simulink model "Motor_Servo_Final"  (R2026a)
settings: Solver=VariableStepAuto  StopTime=10
values from neighbouring files (symbols this model uses):
  b = 0.1    [parameters.m]
  J = 0.01    [parameters.m]
  K = Ka(1:2)    [observer_design.m]    (also in servo_controller.m; state_feedback.m = place(A,B,desired_poles))
  Ke = 0.01    [parameters.m]
  Ki = -Ka(3)    [observer_design.m]    (also in servo_controller.m = Ka(3))
  Kt = 0.01    [parameters.m]
  L = 0.5    [observer_design.m]    (also in parameters.m)
  R = 1    [parameters.m]
settings Model: Creator=DELL  LastModifiedBy=DELL

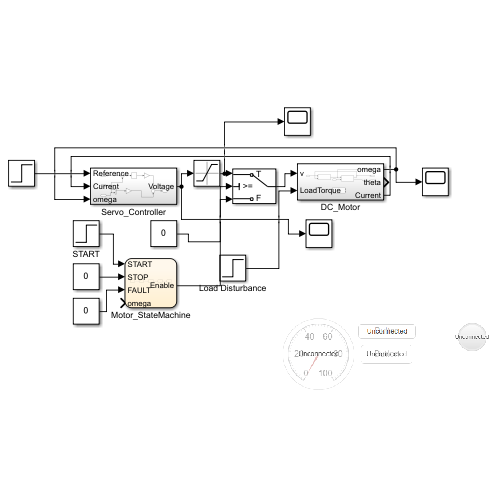
[thumbnail: Simulink's stored preview of the top-level diagram]
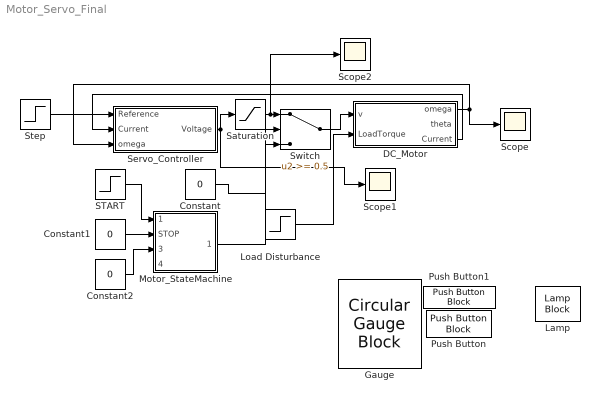
== system Motor_Servo_Final ==
  Constant : Constant  Value=0
  Constant1 : Constant  Value=0
  Constant2 : Constant  Value=0
  DC_Motor : Subsystem
  Gauge : CircularGaugeBlock  FontColor=[0.0, 0.0, 0.0]
  Lamp : LampBlock  LabelPosition=Hide  DefaultColor=[192.0, 192.0, 192.0]
  Load Disturbance : Step  Time=2  FinalValue=0.02  SampleTime=0
  Motor_StateMachine : Stateflow chart  TreatAsAtomicUnit=on
  Push Button : PushButtonBlock  IconOnColor=[0.0, 0.39215686274509803, 0.0]  IconOffColor=[0.0, 1.0, 0.0]
  Push Button1 : PushButtonBlock  IconOnColor=[0.0, 0.39215686274509803, 0.0]  IconOffColor=[0.0, 1.0, 0.0]
  START : Step  Time=0  SampleTime=0
  Saturation : Saturate  UpperLimit=220  LowerLimit=-220
  Scope : Scope
      settings: ActiveDisplayYMinimum=-0.091246608325466383  ActiveDisplayYMaximum=1.905925597827455
  Scope1 : Scope
      settings: ActiveDisplayYMinimum=-1002.8339969118642  ActiveDisplayYMaximum=2013.0889387942134
  Scope2 : Scope
      settings: ActiveDisplayYMinimum=-27.499999999999993  ActiveDisplayYMaximum=247.5  DataLoggingVariableName=ScopeData2
  Servo_Controller : Subsystem
  Step : Step  Time=0  FinalValue=10  SampleTime=0
  Switch : Switch  Threshold=0.5  SaturateOnIntegerOverflow=off  InputSameDT=off
  wires:
  DC_Motor/1(omega) -> Scope/1, Servo_Controller/3(omega)
  Load Disturbance/1 -> DC_Motor/2(LoadTorque)
  DC_Motor/3(Current) -> Servo_Controller/2(Current)
  Constant/1 -> Switch/3
  START/1 -> Motor_StateMachine/1(START)
  Constant1/1 -> Motor_StateMachine/2(STOP)
  Constant2/1 -> Motor_StateMachine/3(FAULT)
  Step/1 -> Servo_Controller/1(Reference)
  Motor_StateMachine/1(Enable) -> Switch/2
  Switch/1 -> DC_Motor/1(v)
  Servo_Controller/1(Voltage) -> Saturation/1, Scope1/1
  Saturation/1 -> Scope2/1, Switch/1

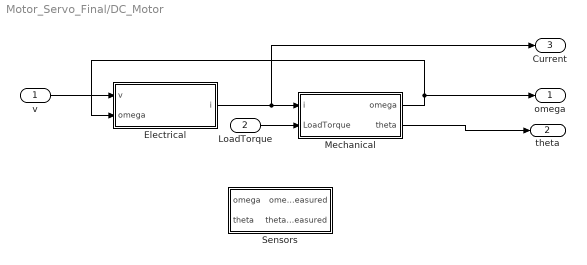
== system Motor_Servo_Final/DC_Motor ==
  v : Inport
  LoadTorque : Inport  Port=2
  Electrical : Subsystem
  Mechanical : Subsystem
  Sensors : Subsystem
  omega : Outport
  theta : Outport  Port=2
  Current : Outport  Port=3
  wires:
  v/1 -> Electrical/1(v)
  Mechanical/1(omega) -> Electrical/2(omega), omega/1
  Mechanical/2(theta) -> theta/1
  LoadTorque/1 -> Mechanical/2(LoadTorque)
  Electrical/1(i) -> Current/1, Mechanical/1(i)

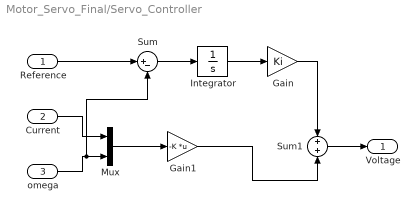
== system Motor_Servo_Final/Servo_Controller ==
  Reference : Inport
  Current : Inport  Port=2
  omega : Inport  Port=3
  Gain : Gain  Gain=Ki
  Gain1 : Gain  Gain=-K  Multiplication=Matrix(K*u)
  Integrator : Integrator
  Mux : Mux  Inputs=2
  Sum : Sum  Inputs=|+-
  Sum1 : Sum
  Voltage : Outport
  wires:
  omega/1 -> Sum/2, Mux/2
  Current/1 -> Mux/1
  Reference/1 -> Sum/1
  Sum/1 -> Integrator/1
  Integrator/1 -> Gain/1
  Mux/1 -> Gain1/1
  Gain/1 -> Sum1/1
  Gain1/1 -> Sum1/2
  Sum1/1 -> Voltage/1

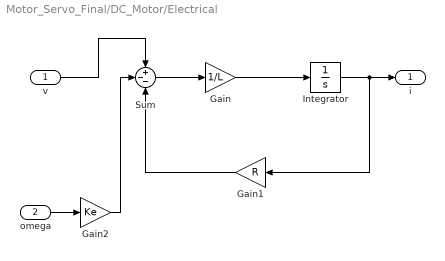
== system Motor_Servo_Final/DC_Motor/Electrical ==
  v : Inport
  omega : Inport  Port=2
  Gain : Gain  Gain=1/L
  Gain1 : Gain  Gain=R
  Gain2 : Gain  Gain=Ke
  Integrator : Integrator
  Sum : Sum  Inputs=+--
  i : Outport
  wires:
  v/1 -> Sum/1
  Sum/1 -> Gain/1
  Gain/1 -> Integrator/1
  Integrator/1 -> Gain1/1, i/1
  omega/1 -> Gain2/1
  Gain1/1 -> Sum/3
  Gain2/1 -> Sum/2

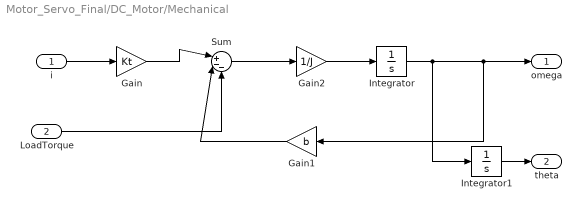
== system Motor_Servo_Final/DC_Motor/Mechanical ==
  i : Inport
  LoadTorque : Inport  Port=2
  Gain : Gain  Gain=Kt
  Gain1 : Gain  Gain=b
  Gain2 : Gain  Gain=1/J
  Integrator : Integrator
  Integrator1 : Integrator
  Sum : Sum  Inputs=|+--
  omega : Outport
  theta : Outport  Port=2
  wires:
  i/1 -> Gain/1
  Gain/1 -> Sum/1
  Sum/1 -> Gain2/1
  Gain2/1 -> Integrator/1
  Integrator/1 -> Integrator1/1, Gain1/1, omega/1
  Gain1/1 -> Sum/2
  Integrator1/1 -> theta/1
  LoadTorque/1 -> Sum/3

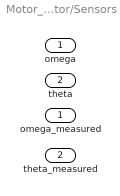
== system Motor_Servo_Final/DC_Motor/Sensors ==
  omega : Inport
  theta : Inport  Port=2
  omega_measured : Outport
  theta_measured : Outport  Port=2

== stateflow chart Motor_Servo_Final/Motor_StateMachine ==
  state OFF
    entry:
    Enable=0;
  state START
    entry:
    Enable=1;
  state ACCELERATION
    during:
    Enable=1;
  state RUNNING
    during:
    Enable=1;
  state STOP
    entry:
    Enable=0;
  state FAULT
    entry:
    Enable=0;
  (default) -> OFF
  OFF -> START : [START==1]
  START -> ACCELERATION : after(1,sec)
  ACCELERATION -> RUNNING : [omega>=9.8]
  RUNNING -> STOP [order 1] : [STOP==1]
  RUNNING -> FAULT [order 2] : [FAULT==1]
  STOP -> FAULT : after(1,sec)
  data: START input; STOP input; FAULT input; Enable output; omega input
